simulink model "sm_car_testrig_bus_VehBusBrakes"  (R2018b)
settings: Solver=VariableStepAuto  StartTime=0.0  StopTime=10.0  RelTol=1e-3
libraries: fl_lib x8, sm_car_lib x4, nesl_utility x1
Description:
  | Copyright 2020 The MathWorks, Inc.
settings Model: Creator=smiller  LastModifiedBy=smiller
settings ExplorerConfigSet: SimMechanicsOpenEditorOnUpdate=off

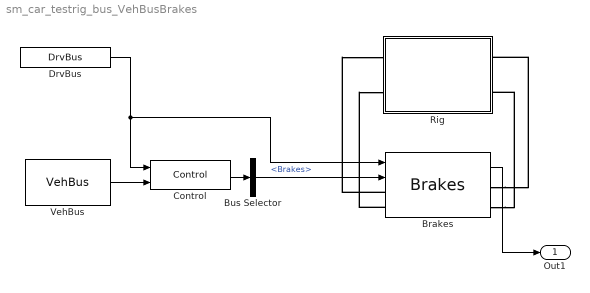
== system sm_car_testrig_bus_VehBusBrakes ==
  Brakes : sm_car_lib/Brakes/Brakes  Tag=PublishSubsystem  VariantControl=Variant1  Brakes=Vehicle.Brakes  VariantLabel=Vehicle.Brakes.class.Value  InitTriggerDropdown=1
      settings: AttributesFormatString=%<ActiveVariant>
  Bus Selector : BusSelector  OutputSignals=Brakes
  Control : sm_car_lib/Control/Control  popup_brake_control=Pedal  trq_ratio_front=1
      settings: AttributesFormatString=%<popup_brake_control>
  DrvBus : sm_car_lib/Inputs/DrvBus  SystemSampleTime=-1
  Rig : Subsystem
  VehBus : sm_car_lib/Outputs/VehBus  SystemSampleTime=-1
  Out1 : Outport  OutDataTypeStr=Bus: VehicleBrakesBusDef
      settings: AttributesFormatString=%<OutDataTypeStr>
  wires:
  Brakes/1 -> Out1/1
  Bus Selector/1 -> Brakes/2  "<Brakes>"
  Control/1 -> Bus Selector/1
  DrvBus/1 -> Control/1, Brakes/1
  VehBus/1 -> Control/2
  connections:
  Brakes/LConn1 -- Rig/LConn1
  Brakes/RConn1 -- Rig/RConn1
  Brakes/RConn2 -- Rig/RConn2
  Brakes/LConn2 -- Rig/LConn2

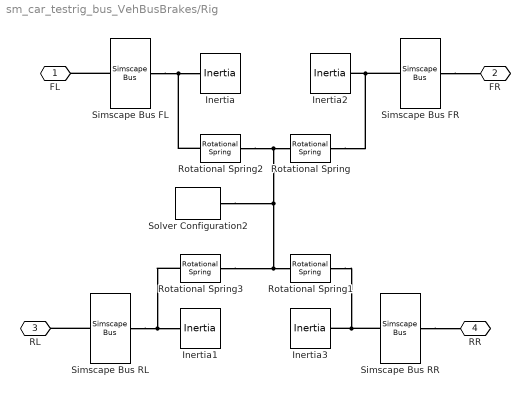
== system sm_car_testrig_bus_VehBusBrakes/Rig ==
  Inertia{,1..3} (4 alike) : fl_lib/Mechanical/Rotational Elements/Inertia  inertia=0.01 kg*m^2  w_specify=off  w_priority=High  w=0 rad/s  w_nominal_specify=off  w_nominal_unit=rad/s  w_nominal_value=1  t_specify=off  t_priority=None  t=0 N*m  t_nominal_specify=off  t_nominal_unit=N*m  t_nominal_value=1
  Rotational Spring{,1..3} (4 alike) : fl_lib/Mechanical/Rotational Elements/Rotational Spring  spr_rate=10 N*m/rad  w_specify=off  w_priority=None  w=0 rad/s  w_nominal_specify=off  w_nominal_unit=rad/s  w_nominal_value=1  t_specify=off  t_priority=None  t=0 N*m  t_nominal_specify=off  t_nominal_unit=N*m  t_nominal_value=1  phi_specify=off  phi_priority=High  phi=0 rad  phi_nominal_specify=off  phi_nominal_unit=rad  phi_nominal_value=1
      settings: SourceProductName=Simscape
  Simscape Bus FL : SimscapeBus  HierarchyStrings=Axle1D
  Simscape Bus FR : SimscapeBus  HierarchyStrings=Axle1D
  Simscape Bus RL : SimscapeBus  HierarchyStrings=Axle1D
  Simscape Bus RR : SimscapeBus  HierarchyStrings=Axle1D
  Solver Configuration2 : nesl_utility/Solver Configuration  PhysicalDomain=network_engine_domain  SubClassName=solver  LeftPortType=input  RightPortType=generic  Tones=[]  Harmonics=[]  SimulateNoise=off  Profile=off  UseLocalSampling=off  EnableSwitchedLinearOptims=on  FrequencyDomain=off  UseCCode=off  RelTol=0.001  AbsTol=1e-06  MinStep=1e-09  ToWorkspace=off  RevertToSquareIcSolve=off  NumHomotopyIterations=100  PhasorMode=off  PhasorModeNumHarmonics=1  DoDC=off  ResidualTolerance=1e-09  UseLocalSolver=off  LocalSolverChoice=NE_BACKWARD_EULER_ADVANCER  LocalSolverSampleTime=0.001  DoFixedCost=off  MaxNonlinIter=3  MaxModeIter=2  LinearAlgebra=auto  EquationFormulation=NE_TIME_EF  DelaysMemoryBudget=1024  AutomaticFiltering=on  FilteringTimeConstant=0.001  PartitionStorageMethod=AS_NEEDED  PartitionMemoryBudget=1024
  FL : PMIOPort  Side=Left
  FR : PMIOPort  Port=2  Side=Right
  RL : PMIOPort  Port=3  Side=Left
  RR : PMIOPort  Port=4  Side=Right
  connections:
  Simscape Bus FL/RConn1 -- FL/RConn1
  Simscape Bus FR/RConn1 -- FR/RConn1
  Simscape Bus RL/RConn1 -- RL/RConn1
  Simscape Bus RR/RConn1 -- RR/RConn1
  Simscape Bus FL/LConn1 -- Rotational Spring2/RConn1 -- Inertia/LConn1
  Simscape Bus RL/LConn1 -- Rotational Spring3/RConn1 -- Inertia1/LConn1
  Simscape Bus FR/LConn1 -- Rotational Spring/RConn1 -- Inertia2/LConn1
  Simscape Bus RR/LConn1 -- Rotational Spring1/RConn1 -- Inertia3/LConn1
  Rotational Spring2/LConn1 -- Solver Configuration2/RConn1 -- Rotational Spring1/LConn1 -- Rotational Spring3/LConn1 -- Rotational Spring/LConn1
